simulink library "Airframes"  (Simulink 7.3)
settings: Solver=ode45  StartTime=0.0  StopTime=10.0  RelTol=1e-3
undefined symbols (not defined in the file or in its folder): Vo
libraries: aero_sim_lib x4, simulink x2
(part 2 of 2)

== system Airframes/Cesna A-37/T-37Airframe/Aero. Coef. (Stability Axis)/[C_Y,C_g_L,C_g_N] ==
  u : Inport
  CY_p : Constant  Value=CY_p  OutDataType=fixdt(1, 16)  OutScaling=2^0
  Clm_p : Constant  Value=Clm_p  OutDataType=fixdt(1, 16)  OutScaling=2^0
  Cmm_p : Constant  Value=Cnm_p  OutDataType=fixdt(1, 16)  OutScaling=2^0
  Dot Product : DotProduct  OutDataType=fixdt(1, 16)  OutScaling=2^-10  InputSameDT=on  OutDataTypeStr=Inherit: Inherit via internal rule
  Dot Product1 : DotProduct  OutDataType=fixdt(1, 16)  OutScaling=2^-10  InputSameDT=on  OutDataTypeStr=Inherit: Inherit via internal rule
  Dot Product2 : DotProduct  OutDataType=fixdt(1, 16)  OutScaling=2^-10  InputSameDT=on  OutDataTypeStr=Inherit: Inherit via internal rule
  C_Y : Outport
  C_g_L : Outport  Port=2
  C_g_N : Outport  Port=3
  wires:
  Dot Product2/1 -> C_g_N/1  "C_g_N"
  Dot Product1/1 -> C_g_L/1  "C_g_L"
  Dot Product/1 -> C_Y/1  "C_Y"
  Cmm_p/1 -> Dot Product2/2
  CY_p/1 -> Dot Product/2
  u/1 -> Dot Product/1, Dot Product1/1, Dot Product2/1
  Clm_p/1 -> Dot Product1/2

== system Airframes/Cesna A-37/T-37Airframe/Alpha,Beta,Mach/Dynamic Pressure ==
  V : Inport  OutDataType=sfix(16)  OutScaling=2^0
  Air Density : Inport  Port=2  OutDataType=sfix(16)  OutScaling=2^0
  1/2rhoV^2 : Gain  Gain=1/2  ParameterDataType=sfix(16)  ParameterScaling=2^0  OutDataType=sfix(16)  OutScaling=2^0  SaturateOnIntegerOverflow=on  OutDataTypeStr=Inherit: Same as input  ParamDataTypeStr=Inherit: Same as input
  Product1 : Product  OutDataType=sfix(16)  OutScaling=2^0  SaturateOnIntegerOverflow=on  InputSameDT=on  OutDataTypeStr=Inherit: Same as first input
  Product2 : Product  OutDataType=sfix(16)  OutScaling=2^0  SaturateOnIntegerOverflow=on  InputSameDT=on  OutDataTypeStr=Inherit: Same as first input
  qbar : Outport  OutDataType=sfix(16)  OutScaling=2^0  InitialOutput=0
  wires:
  1/2rhoV^2/1 -> qbar/1
  Product2/1 -> 1/2rhoV^2/1
  Air Density/1 -> Product2/2
  Product1/1 -> Product2/1
  V/1 -> Product1/1, Product1/2

== system Airframes/Cesna A-37/T-37Airframe/Alpha,Beta,Mach/Incidence, Sideslip & Airspeed ==
  Vb : Inport  OutDataType=sfix(16)  OutScaling=2^0
  Airspeed : Math  Operator=sqrt  OutDataType=sfix(16)  OutScaling=2^0  SaturateOnIntegerOverflow=on
  Dot Product : DotProduct  OutDataType=fixdt(1, 16)  OutScaling=2^-10  InputSameDT=on  OutDataTypeStr=Inherit: Inherit via internal rule
  Incidence : Trigonometry  Operator=atan2
  Product : Product  Inputs=*/  OutDataType=sfix(16)  OutScaling=2^0  SaturateOnIntegerOverflow=on  OutDataTypeStr=Inherit: Same as first input
  Sideslip : Trigonometry  Operator=asin
  Subsystem : Subsystem
  Subsystem1 : Subsystem
  Alpha : Outport  OutDataType=sfix(16)  OutScaling=2^0  InitialOutput=0
  Beta : Outport  Port=2  OutDataType=sfix(16)  OutScaling=2^0  InitialOutput=0
  V : Outport  Port=3  OutDataType=sfix(16)  OutScaling=2^0  InitialOutput=0
  wires:
  Product/1 -> Sideslip/1
  Subsystem/1(w) -> Incidence/1
  Subsystem/2(u) -> Incidence/2
  Dot Product/1 -> Airspeed/1
  Airspeed/1 -> Product/2, V/1
  Incidence/1 -> Alpha/1
  Vb/1 -> Subsystem/1(Vb), Subsystem1/1(Vb), Dot Product/1, Dot Product/2
  Sideslip/1 -> Beta/1
  Subsystem1/1(v) -> Product/1

== system Airframes/Cesna A-37/T-37Airframe/Alpha,Beta,Mach/Mach Number ==
  V : Inport  OutDataType=sfix(16)  OutScaling=2^0
  a : Inport  Port=2  OutDataType=sfix(16)  OutScaling=2^0
  Product1 : Product  Inputs=*/  OutDataType=sfix(16)  OutScaling=2^0  SaturateOnIntegerOverflow=on  InputSameDT=on  OutDataTypeStr=Inherit: Same as first input
  Mach : Outport  OutDataType=sfix(16)  OutScaling=2^0
  wires:
  Product1/1 -> Mach/1
  a/1 -> Product1/2
  V/1 -> Product1/1

== system Airframes/Cesna A-37/T-37Airframe/Environment Models/Wind Models ==
  Euler : Inport  OutDataType=sfix(16)  OutScaling=2^0
  Ve : Inport  Port=2  OutDataType=sfix(16)  OutScaling=2^0
  Airspeed : Inport  Port=3  OutDataType=sfix(16)  OutScaling=2^0
  Altitude : Inport  Port=4  OutDataType=sfix(16)  OutScaling=2^0
  DCM : Inport  Port=5  OutDataType=sfix(16)  OutScaling=2^0
  MIL-F-8785C Wind Gust Model (to do) : Subsystem  mask{G_u=on, G_v=on, G_w=on, t_0=100, x_m=10*[b,b,b], v_m=[5,5,5]}
      mask prompts: G_u "Gust in u-axis [G_u]"; G_v "Gust in v-axis [G_v]"; G_w "Gust in w-axis [G_w]"; t_0 "Gust start-time [t_0] (sec):"; x_m "Gust legth x_m=[x_u,x_v,x_w] (m):"; v_m "Gust amplitude v_m=[v_u,v_v,v_w](m/s):"
  MIL-F-8785C Wind Shear Model : Subsystem  mask{phase=Category C (Terminal Flight), u20=6, deg=0}
      mask prompts: phase "Select Flight Phase [phase]"; u20 "Wind Speed at 20 feet above ground [u20] (m/sec)"; deg "Approach Angle of Wind (clock-wise from the North) [deg] (degrees)"
      mask StyleString: popup(Category C (Terminal Flight)|Category A or B (Not Terminal Flight)),edit,edit
  Need Dryden Turbulent Model Block : Constant  Value=[0,0,0]  OutDataType=fixdt(1, 16)  OutScaling=2^0
  Sum : Sum  Inputs=+|+  OutDataType=sfix(16)  OutScaling=2^0  SaturateOnIntegerOverflow=on  InputSameDT=on  OutDataTypeStr=Inherit: Same as first input
  Terminator : Terminator
  Terminator1 : Terminator
  ug,vg,wg : Outport  OutDataType=sfix(16)  OutScaling=2^0
  pg,qg,rg : Outport  Port=2  OutDataType=sfix(16)  OutScaling=2^0
  wires:
  Altitude/1 -> MIL-F-8785C Wind Shear Model/1(h)
  Airspeed/1 -> MIL-F-8785C Wind Gust Model (to do)/1(V(m/s))
  DCM/1 -> MIL-F-8785C Wind Shear Model/2(DCM)
  Sum/1 -> ug,vg,wg/1
  Ve/1 -> Terminator/1
  Euler/1 -> Terminator1/1
  MIL-F-8785C Wind Shear Model/1(v_w) -> Sum/1
  MIL-F-8785C Wind Gust Model (to do)/1(v_w(m/s)) -> Sum/2
  Need Dryden Turbulent Model Block/1 -> pg,qg,rg/1

== system Airframes/Cesna A-37/T-37Airframe/Environment Models/gravity model ==
  h : Inport
  Divide : Product  Inputs=*/  OutDataType=fixdt(1, 16)  OutScaling=2^-10
  Dot Product1 : DotProduct  OutDataType=fixdt(1, 16)  OutScaling=2^-10  InputSameDT=on  OutDataTypeStr=Inherit: Inherit via internal rule
  Model Info : simulink/Model-Wide Utilities/Model Info  SystemSampleTime=-1  InitialBlockCM=None  BlockCM=None  Frame=on  DisplayStringWithTags=g = g_o [R/(R+h)]^2  HorizontalTextAlignment=Center  LeftAlignmentValue=0.5  SourceBlockDiagram=Airframes  TagMaxNumber=20
  R = Radius of Earth (m) : Constant  Value=6356e3  OutDataType=fixdt(1, 16)  OutScaling=2^0
  Sum : Sum  Inputs=|++  OutDataType=fixdt(1, 16)  OutScaling=2^0
  g_o : Gain  Gain=9.80665  ParameterDataType=fixdt(1, 16)  ParameterScaling=2^0  OutDataType=fixdt(1, 16)  OutScaling=2^0
  g : Outport
  wires:
  R = Radius of Earth (m)/1 -> Sum/2, Divide/1
  Sum/1 -> Divide/2
  Divide/1 -> Dot Product1/1, Dot Product1/2
  Dot Product1/1 -> g_o/1
  h/1 -> Sum/1
  g_o/1 -> g/1

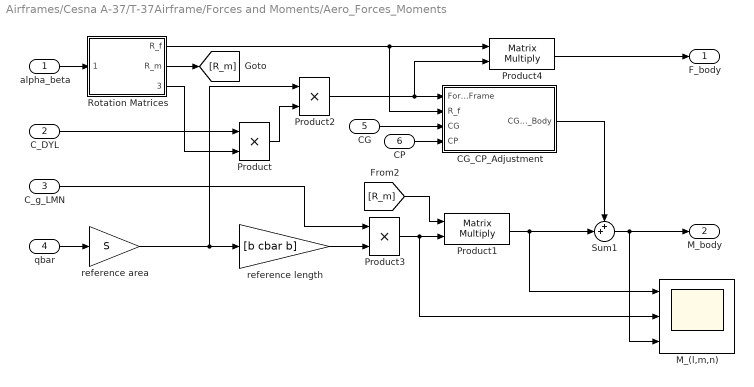
== system Airframes/Cesna A-37/T-37Airframe/Forces and Moments/Aero_Forces_Moments ==
  alpha_beta : Inport
  C_DYL : Inport  Port=2
  C_g_LMN : Inport  Port=3
  qbar : Inport  Port=4
  CG : Inport  Port=5  OutDataType=sfix(16)  OutScaling=2^0
  CP : Inport  Port=6  OutDataType=sfix(16)  OutScaling=2^0
  CG_CP_Adjustment : Subsystem
  M_(l,m,n) : Scope  NumInputPorts=3
      settings: YMin=-5~-5~-5  YMax=5~5~5  SaveName=ScopeData7  SampleInput=on  SampleTime=0.01
  Product : Product  OutDataType=sfix(16)  OutScaling=2^0  SaturateOnIntegerOverflow=on  InputSameDT=on  OutDataTypeStr=Inherit: Same as first input
  Product1 : Product  Multiplication=Matrix(*)  OutDataType=sfix(16)  OutScaling=2^0  RndMeth=Zero
  Product2 : Product  OutDataType=sfix(16)  OutScaling=2^0  SaturateOnIntegerOverflow=on  InputSameDT=on  OutDataTypeStr=Inherit: Same as first input
  Product3 : Product  OutDataType=sfix(16)  OutScaling=2^0  SaturateOnIntegerOverflow=on  InputSameDT=on  OutDataTypeStr=Inherit: Same as first input
  Product4 : Product  Multiplication=Matrix(*)  OutDataType=sfix(16)  OutScaling=2^0  RndMeth=Zero
  Rotation Matrices : Stateflow chart
  Sum1 : Sum  Inputs=++|  OutDataType=sfix(16)  OutScaling=2^0  SaturateOnIntegerOverflow=on  InputSameDT=on  OutDataTypeStr=Inherit: Same as first input
  reference area : Gain  Gain=S  ParameterDataType=sfix(16)  ParameterScaling=2^0  OutDataType=sfix(16)  OutScaling=2^0  SaturateOnIntegerOverflow=on  OutDataTypeStr=Inherit: Same as input  ParamDataTypeStr=Inherit: Same as input
  reference length : Gain  Gain=[b cbar b]  ParameterDataType=sfix(16)  ParameterScaling=2^0  OutDataType=sfix(16)  OutScaling=2^0  SaturateOnIntegerOverflow=on  OutDataTypeStr=Inherit: Same as input  ParamDataTypeStr=Inherit: Same as input
  F_body : Outport
  M_body : Outport  Port=2
  wires:
  alpha_beta/1 -> Rotation Matrices/1(alpha_beta)
  qbar/1 -> reference area/1
  reference area/1 -> reference length/1, Product2/1
  C_DYL/1 -> Product/1
  Rotation Matrices/3(K_adjust) -> Product/2
  reference length/1 -> Product3/2
  C_g_LMN/1 -> Product3/1
  CG/1 -> CG_CP_Adjustment/3(CG)
  CP/1 -> CG_CP_Adjustment/4(CP)
  Rotation Matrices/1(R_f) -> Product4/1, CG_CP_Adjustment/2(R_f)
  Product/1 -> Product2/2
  Product2/1 -> Product4/2, CG_CP_Adjustment/1(Forces_Drag_Frame)
  Product4/1 -> F_body/1
  Rotation Matrices/2(R_m) -> [R_m]
  [R_m] -> Product1/1
  Product3/1 -> M_(l,m,n)/2, Product1/2
  Product1/1 -> M_(l,m,n)/1, Sum1/2
  CG_CP_Adjustment/1(CGP_M_Body) -> Sum1/1
  Sum1/1 -> M_(l,m,n)/3, M_body/1

== system Airframes/Cesna 172P (Skyhawk) Airframe/Alpha,Beta,Mach/Incidence, Sideslip & Airspeed/Subsystem ==
  Vb : Inport  OutDataType=sfix(16)  OutScaling=2^0
  Demux1 : Demux  Outputs=3
  Terminator : Terminator
  w : Outport  OutDataType=sfix(16)  OutScaling=2^0
  u : Outport  Port=2  OutDataType=sfix(16)  OutScaling=2^0
  wires:
  Demux1/1 -> u/1
  Vb/1 -> Demux1/1
  Demux1/2 -> Terminator/1
  Demux1/3 -> w/1

== system Airframes/Cesna 172P (Skyhawk) Airframe/Alpha,Beta,Mach/Incidence, Sideslip & Airspeed/Subsystem1 ==
  Vb : Inport  OutDataType=sfix(16)  OutScaling=2^0
  Demux1 : Demux  Outputs=3
  Terminator : Terminator
  Terminator1 : Terminator
  v : Outport  OutDataType=sfix(16)  OutScaling=2^0
  wires:
  Demux1/2 -> v/1
  Vb/1 -> Demux1/1
  Demux1/3 -> Terminator1/1
  Demux1/1 -> Terminator/1

== system Airframes/Cesna 172P (Skyhawk) Airframe/Environment Models/Wind Models/MIL-F-8785C Wind Gust Model (to do) ==
  V(m/s) : Inport
  Clock : Clock
      settings: Decimation=10
  Constant : Constant  Value=t_0  OutDataType=fixdt(1, 16)  OutScaling=2^0
  Relational Operator : RelationalOperator  LogicOutDataTypeMode=boolean  LogicDataType=fixdt(0, 8)  OutDataTypeStr=boolean
  Triggered Gusts : Subsystem
  v_w(m/s) : Outport
  wires:
  Triggered Gusts/1(v_w) -> v_w(m/s)/1
  V(m/s)/1 -> Triggered Gusts/1(V(m/s))
  Relational Operator/1 -> Triggered Gusts/Enable
  Constant/1 -> Relational Operator/2
  Clock/1 -> Relational Operator/1

== system Airframes/Cesna 172P (Skyhawk) Airframe/Environment Models/Wind Models/MIL-F-8785C Wind Shear Model ==
  h : Inport
  DCM : Inport  Port=2
  MIL-F-8785-Wind Shear Model : Stateflow chart
  v_w : Outport
  wires:
  MIL-F-8785-Wind Shear Model/1(v_w) -> v_w/1
  DCM/1 -> MIL-F-8785-Wind Shear Model/2(DCM)
  h/1 -> MIL-F-8785-Wind Shear Model/1(h)

== system Airframes/Cesna 172P (Skyhawk) Airframe/Forces and Moments/Aero_Forces_Moments/CG_CP_Adjustment ==
  Forces_Drag_Frame : Inport
  R_f : Inport  Port=2
  CG : Inport  Port=3
  CP : Inport  Port=4
  CrossProduct(AXB) : aero_sim_lib/CrossProduct(AXB)  SystemSampleTime=-1
  Product1 : Product  Multiplication=Matrix(*)  OutDataType=sfix(16)  OutScaling=2^0  RndMeth=Zero
  Product2 : Product  Multiplication=Matrix(*)  OutDataType=sfix(16)  OutScaling=2^0  RndMeth=Zero
  Sum : Sum  Inputs=|+-  OutDataType=sfix(16)  OutScaling=2^0  SaturateOnIntegerOverflow=on
  Transpose : Math  Operator=transpose  OutDataType=sfix(16)  OutScaling=2^0  SaturateOnIntegerOverflow=on
  CGP_M_Body : Outport
  wires:
  CrossProduct(AXB)/1 -> Product2/2  "CGP_Moments_Drag_Frame"
  Product2/1 -> CGP_M_Body/1
  CP/1 -> Sum/2
  CG/1 -> Sum/1
  R_f/1 -> Product2/1, Transpose/1  "Rotation_Matrix_Drag_Frame_To_Body_Frame"
  Forces_Drag_Frame/1 -> CrossProduct(AXB)/1
  Product1/1 -> CrossProduct(AXB)/2  "DX_Drag_Frame"
  Sum/1 -> Product1/2  "DX_Body"
  Transpose/1 -> Product1/1

== system Airframes/Cesna A-37/T-37Airframe/Alpha,Beta,Mach/Incidence, Sideslip & Airspeed/Subsystem ==
  Vb : Inport  OutDataType=sfix(16)  OutScaling=2^0
  Demux1 : Demux  Outputs=3
  Terminator : Terminator
  w : Outport  OutDataType=sfix(16)  OutScaling=2^0
  u : Outport  Port=2  OutDataType=sfix(16)  OutScaling=2^0
  wires:
  Demux1/3 -> w/1
  Demux1/2 -> Terminator/1
  Vb/1 -> Demux1/1
  Demux1/1 -> u/1

== system Airframes/Cesna A-37/T-37Airframe/Alpha,Beta,Mach/Incidence, Sideslip & Airspeed/Subsystem1 ==
  Vb : Inport  OutDataType=sfix(16)  OutScaling=2^0
  Demux1 : Demux  Outputs=3
  Terminator : Terminator
  Terminator1 : Terminator
  v : Outport  OutDataType=sfix(16)  OutScaling=2^0
  wires:
  Demux1/1 -> Terminator/1
  Demux1/3 -> Terminator1/1
  Vb/1 -> Demux1/1
  Demux1/2 -> v/1

== system Airframes/Cesna A-37/T-37Airframe/Environment Models/Wind Models/MIL-F-8785C Wind Gust Model (to do) ==
  V(m/s) : Inport
  Clock : Clock
      settings: Decimation=10
  Constant : Constant  Value=t_0  OutDataType=fixdt(1, 16)  OutScaling=2^0
  Relational Operator : RelationalOperator  LogicOutDataTypeMode=boolean  LogicDataType=fixdt(0, 8)  OutDataTypeStr=boolean
  Triggered Gusts : Subsystem
  v_w(m/s) : Outport
  wires:
  Clock/1 -> Relational Operator/1
  Constant/1 -> Relational Operator/2
  Relational Operator/1 -> Triggered Gusts/Enable
  V(m/s)/1 -> Triggered Gusts/1(V(m/s))
  Triggered Gusts/1(v_w) -> v_w(m/s)/1

== system Airframes/Cesna A-37/T-37Airframe/Environment Models/Wind Models/MIL-F-8785C Wind Shear Model ==
  h : Inport
  DCM : Inport  Port=2
  MIL-F-8785-Wind Shear Model : Stateflow chart
  v_w : Outport
  wires:
  h/1 -> MIL-F-8785-Wind Shear Model/1(h)
  DCM/1 -> MIL-F-8785-Wind Shear Model/2(DCM)
  MIL-F-8785-Wind Shear Model/1(v_w) -> v_w/1

== system Airframes/Cesna A-37/T-37Airframe/Forces and Moments/Aero_Forces_Moments/CG_CP_Adjustment ==
  Forces_Drag_Frame : Inport
  R_f : Inport  Port=2
  CG : Inport  Port=3
  CP : Inport  Port=4
  CrossProduct(AXB) : aero_sim_lib/CrossProduct(AXB)  SystemSampleTime=-1
  Product1 : Product  Multiplication=Matrix(*)  OutDataType=sfix(16)  OutScaling=2^0  RndMeth=Zero
  Product2 : Product  Multiplication=Matrix(*)  OutDataType=sfix(16)  OutScaling=2^0  RndMeth=Zero
  Sum : Sum  Inputs=|+-  OutDataType=sfix(16)  OutScaling=2^0  SaturateOnIntegerOverflow=on
  Transpose : Math  Operator=transpose  OutDataType=sfix(16)  OutScaling=2^0  SaturateOnIntegerOverflow=on
  CGP_M_Body : Outport
  wires:
  Transpose/1 -> Product1/1
  Sum/1 -> Product1/2  "DX_Body"
  Product1/1 -> CrossProduct(AXB)/2  "DX_Drag_Frame"
  Forces_Drag_Frame/1 -> CrossProduct(AXB)/1
  R_f/1 -> Transpose/1, Product2/1  "Rotation_Matrix_Drag_Frame_To_Body_Frame"
  CG/1 -> Sum/1
  CP/1 -> Sum/2
  Product2/1 -> CGP_M_Body/1
  CrossProduct(AXB)/1 -> Product2/2  "CGP_Moments_Drag_Frame"

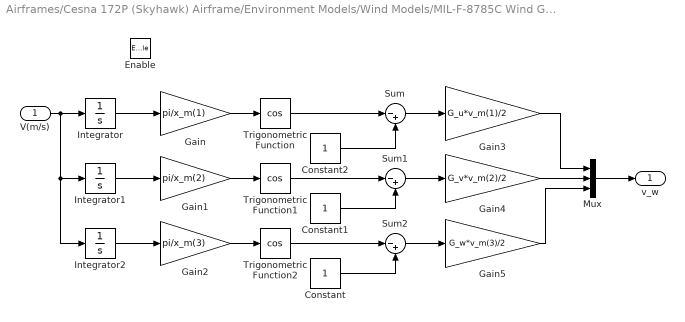
== system Airframes/Cesna 172P (Skyhawk) Airframe/Environment Models/Wind Models/MIL-F-8785C Wind Gust Model (to do)/Triggered Gusts ==
  V(m/s) : Inport
  Enable : EnablePort
  Constant : Constant  OutDataType=fixdt(1, 16)  OutScaling=2^0
  Constant1 : Constant  OutDataType=fixdt(1, 16)  OutScaling=2^0
  Constant2 : Constant  OutDataType=fixdt(1, 16)  OutScaling=2^0
  Gain : Gain  Gain=pi/x_m(1)  ParameterDataType=fixdt(1, 16)  ParameterScaling=2^0  OutDataType=fixdt(1, 16)  OutScaling=2^0
  Gain1 : Gain  Gain=pi/x_m(2)  ParameterDataType=fixdt(1, 16)  ParameterScaling=2^0  OutDataType=fixdt(1, 16)  OutScaling=2^0
  Gain2 : Gain  Gain=pi/x_m(3)  ParameterDataType=fixdt(1, 16)  ParameterScaling=2^0  OutDataType=fixdt(1, 16)  OutScaling=2^0
  Gain3 : Gain  Gain=G_u*v_m(1)/2  ParameterDataType=fixdt(1, 16)  ParameterScaling=2^0  OutDataType=fixdt(1, 16)  OutScaling=2^0
  Gain4 : Gain  Gain=G_v*v_m(2)/2  ParameterDataType=fixdt(1, 16)  ParameterScaling=2^0  OutDataType=fixdt(1, 16)  OutScaling=2^0
  Gain5 : Gain  Gain=G_w*v_m(3)/2  ParameterDataType=fixdt(1, 16)  ParameterScaling=2^0  OutDataType=fixdt(1, 16)  OutScaling=2^0
  Integrator : Integrator  LimitOutput=on  UpperSaturationLimit=x_m(1)  LowerSaturationLimit=0
  Integrator1 : Integrator  LimitOutput=on  UpperSaturationLimit=x_m(2)  LowerSaturationLimit=0
  Integrator2 : Integrator  LimitOutput=on  UpperSaturationLimit=x_m(3)  LowerSaturationLimit=0
  Mux : Mux  Inputs=3
  Sum : Sum  Inputs=|-+  OutDataType=fixdt(1, 16)  OutScaling=2^0
  Sum1 : Sum  Inputs=|-+  OutDataType=fixdt(1, 16)  OutScaling=2^0
  Sum2 : Sum  Inputs=|-+  OutDataType=fixdt(1, 16)  OutScaling=2^0
  Trigonometric Function : Trigonometry  Operator=cos
  Trigonometric Function1 : Trigonometry  Operator=cos
  Trigonometric Function2 : Trigonometry  Operator=cos
  v_w : Outport  OutDataType=fixdt(1, 16)  OutScaling=2^0  InitialOutput=[0,0,0]
  wires:
  Mux/1 -> v_w/1
  Gain5/1 -> Mux/3
  Gain4/1 -> Mux/2
  Gain3/1 -> Mux/1
  Sum1/1 -> Gain4/1
  Sum2/1 -> Gain5/1
  Sum/1 -> Gain3/1
  Constant2/1 -> Sum/2
  Constant1/1 -> Sum1/2
  Constant/1 -> Sum2/2
  Trigonometric Function2/1 -> Sum2/1
  Trigonometric Function1/1 -> Sum1/1
  Trigonometric Function/1 -> Sum/1
  Gain2/1 -> Trigonometric Function2/1
  Integrator2/1 -> Gain2/1
  Gain1/1 -> Trigonometric Function1/1
  Integrator1/1 -> Gain1/1
  Gain/1 -> Trigonometric Function/1
  Integrator/1 -> Gain/1
  V(m/s)/1 -> Integrator2/1, Integrator1/1, Integrator/1

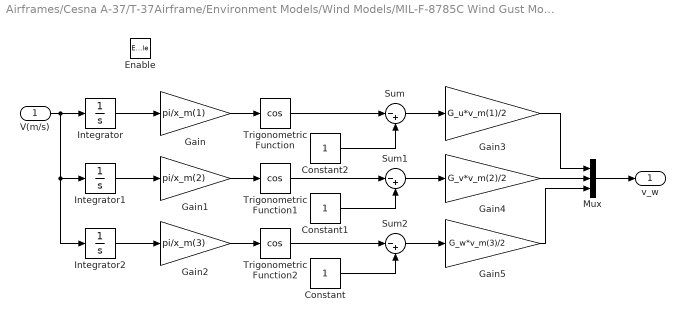
== system Airframes/Cesna A-37/T-37Airframe/Environment Models/Wind Models/MIL-F-8785C Wind Gust Model (to do)/Triggered Gusts ==
  V(m/s) : Inport
  Enable : EnablePort
  Constant : Constant  OutDataType=fixdt(1, 16)  OutScaling=2^0
  Constant1 : Constant  OutDataType=fixdt(1, 16)  OutScaling=2^0
  Constant2 : Constant  OutDataType=fixdt(1, 16)  OutScaling=2^0
  Gain : Gain  Gain=pi/x_m(1)  ParameterDataType=fixdt(1, 16)  ParameterScaling=2^0  OutDataType=fixdt(1, 16)  OutScaling=2^0
  Gain1 : Gain  Gain=pi/x_m(2)  ParameterDataType=fixdt(1, 16)  ParameterScaling=2^0  OutDataType=fixdt(1, 16)  OutScaling=2^0
  Gain2 : Gain  Gain=pi/x_m(3)  ParameterDataType=fixdt(1, 16)  ParameterScaling=2^0  OutDataType=fixdt(1, 16)  OutScaling=2^0
  Gain3 : Gain  Gain=G_u*v_m(1)/2  ParameterDataType=fixdt(1, 16)  ParameterScaling=2^0  OutDataType=fixdt(1, 16)  OutScaling=2^0
  Gain4 : Gain  Gain=G_v*v_m(2)/2  ParameterDataType=fixdt(1, 16)  ParameterScaling=2^0  OutDataType=fixdt(1, 16)  OutScaling=2^0
  Gain5 : Gain  Gain=G_w*v_m(3)/2  ParameterDataType=fixdt(1, 16)  ParameterScaling=2^0  OutDataType=fixdt(1, 16)  OutScaling=2^0
  Integrator : Integrator  LimitOutput=on  UpperSaturationLimit=x_m(1)  LowerSaturationLimit=0
  Integrator1 : Integrator  LimitOutput=on  UpperSaturationLimit=x_m(2)  LowerSaturationLimit=0
  Integrator2 : Integrator  LimitOutput=on  UpperSaturationLimit=x_m(3)  LowerSaturationLimit=0
  Mux : Mux  Inputs=3
  Sum : Sum  Inputs=|-+  OutDataType=fixdt(1, 16)  OutScaling=2^0
  Sum1 : Sum  Inputs=|-+  OutDataType=fixdt(1, 16)  OutScaling=2^0
  Sum2 : Sum  Inputs=|-+  OutDataType=fixdt(1, 16)  OutScaling=2^0
  Trigonometric Function : Trigonometry  Operator=cos
  Trigonometric Function1 : Trigonometry  Operator=cos
  Trigonometric Function2 : Trigonometry  Operator=cos
  v_w : Outport  OutDataType=fixdt(1, 16)  OutScaling=2^0  InitialOutput=[0,0,0]
  wires:
  V(m/s)/1 -> Integrator/1, Integrator1/1, Integrator2/1
  Integrator/1 -> Gain/1
  Gain/1 -> Trigonometric Function/1
  Integrator1/1 -> Gain1/1
  Gain1/1 -> Trigonometric Function1/1
  Integrator2/1 -> Gain2/1
  Gain2/1 -> Trigonometric Function2/1
  Trigonometric Function/1 -> Sum/1
  Trigonometric Function1/1 -> Sum1/1
  Trigonometric Function2/1 -> Sum2/1
  Constant/1 -> Sum2/2
  Constant1/1 -> Sum1/2
  Constant2/1 -> Sum/2
  Sum/1 -> Gain3/1
  Sum2/1 -> Gain5/1
  Sum1/1 -> Gain4/1
  Gain3/1 -> Mux/1
  Gain4/1 -> Mux/2
  Gain5/1 -> Mux/3
  Mux/1 -> v_w/1

== matlab function Cesna A-37/T-37Airframe/Environment Models/Air Properties ==
  data: h input double; T output double; rho output double; g input double; ps output double; a output double
function [T,rho, ps, a] = fcn(h, g)
    %h altitude (meters)
    %g gravity at h (m/s^2)
    R = 8.31432; %J/(mol-Kelvin)
    M = 28.9644; %gm/mol
    To = 288.15; %standard temperature [Kelvin]
    Po = 101325; %standard pressure [Pa]
    L = 6.5; %Kelvin/km
    gamma = 1.4; %Gas constant for air
    T = To - 1.0e-3*L*h;            %Temperature at h
    ps = Po*(T/To)^((g*M)/(R*L));   %Pressure at h
    rho = ps/((1000*R/M)*T);        %Density at h
    a = sqrt(gamma*(R/(M*1e-3))*T); %speed of sound (m/s)

== matlab function Cesna A-37/T-37Airframe/Environment Models/Wind Models/MIL-F-8785C Wind Shear Model/MIL-F-8785-Wind Shear Model ==
  data: h input double; v_w output double; DCM input double; phase parameter double; u20 parameter double; deg parameter double
function v_w = fcn(h, DCM, phase, u20, deg)
%Wind Shear Model Based on
%MIL-F-8785C p. 51
if phase == 1
    z0 = 0.15; %Catagory C Flight Phase (Terminal Flight)
else
    z0 = 2.0;  %Other Flight Phases (Non-Terminal Flight)
end
h = h*3.2808399; %meters to feet
den = log(20/z0);
num = h/z0;
if num < 1
    num = 1;
end
num = log(num);
u_w = u20*num/den;
v_w = DCM*[-u_w*cos(pi*deg/180),-u_w*sin(pi*deg/180),0]';

== matlab function Cesna A-37/T-37Airframe/Forces and Moments/Aero_Forces_Moments/Rotation Matrices ==
  data: C_D_input_axes parameter double; alpha_beta input double; C_g_L_input_axes parameter double; R_f output double; R_m output double; K_adjust output double
function [R_f, R_m, K_adjust] = fcn(C_D_input_axes, alpha_beta, C_g_L_input_axes)
if C_D_input_axes == 1
    R_f=calc_R(alpha_beta(1),0); %stability-to-body
    K_adjust=[-1,1,-1]';
elseif C_D_input_axes == 2
    R_f=calc_R(alpha_beta(1),alpha_beta(2)); %wind-to-body
    K_adjust=[-1,-1,-1]';
else
    R_f=eye(3); %body-to-body
    K_adjust=[1,1,1]';
end
if C_g_L_input_axes == C_D_input_axes
    R_m = R_f;
elseif C_g_L_input_axes == 1
    R_m = calc_R(alpha_beta(1),0); %stability-to-body
elseif C_g_L_input_axes == 2
    R_m = calc_R(alpha_beta(1),alpha_beta(2)); %wind-to-body
else
    R_m=eye(3); %body-to-body
end


function R = calc_R(alpha,beta)
    c_a=cos(alpha);
    c_b=cos(beta);
    s_a=sin(alpha);
    s_b=sin(beta);
    R=[c_a*c_b,-c_a*s_b,-s_a;s_b,c_b,0;s_a*c_b,-s_a*s_b,c_a];

== matlab function Cesna 172P (Skyhawk) Airframe/Environment Models/Air Properties ==
  data: h input double; T output double; rho output double; g input double; ps output double; a output double
function [T,rho, ps, a] = fcn(h, g)
    %h altitude (meters)
    %g gravity at h (m/s^2)
    R = 8.31432; %J/(mol-Kelvin)
    M = 28.9644; %gm/mol
    To = 288.15; %standard temperature [Kelvin]
    Po = 101325; %standard pressure [Pa]
    L = 6.5; %Kelvin/km
    gamma = 1.4; %Gas constant for air
    T = To - 1.0e-3*L*h;            %Temperature at h
    ps = Po*(T/To)^((g*M)/(R*L));   %Pressure at h
    rho = ps/((1000*R/M)*T);        %Density at h
    a = sqrt(gamma*(R/(M*1e-3))*T); %speed of sound (m/s)

== matlab function Cesna 172P (Skyhawk) Airframe/Environment Models/Wind Models/MIL-F-8785C Wind Shear Model/MIL-F-8785-Wind Shear Model ==
  data: h input double; v_w output double; DCM input double; phase parameter double; u20 parameter double; deg parameter double
function v_w = fcn(h, DCM, phase, u20, deg)
%Wind Shear Model Based on
%MIL-F-8785C p. 51
if phase == 1
    z0 = 0.15; %Catagory C Flight Phase (Terminal Flight)
else
    z0 = 2.0;  %Other Flight Phases (Non-Terminal Flight)
end
h = h*3.2808399; %meters to feet
den = log(20/z0);
num = h/z0;
if num < 1
    num = 1;
end
num = log(num);
u_w = u20*num/den;
v_w = DCM*[-u_w*cos(pi*deg/180),-u_w*sin(pi*deg/180),0]';

== matlab function Cesna 172P (Skyhawk) Airframe/Forces and Moments/Aero_Forces_Moments/Rotation Matrices ==
  data: C_D_input_axes parameter double; alpha_beta input double; C_g_L_input_axes parameter double; R_f output double; R_m output double; K_adjust output double
function [R_f, R_m, K_adjust] = fcn(C_D_input_axes, alpha_beta, C_g_L_input_axes)
if C_D_input_axes == 1
    R_f=calc_R(alpha_beta(1),0); %stability-to-body
    K_adjust=[-1,1,-1]';
elseif C_D_input_axes == 2
    R_f=calc_R(alpha_beta(1),alpha_beta(2)); %wind-to-body
    K_adjust=[-1,-1,-1]';
else
    R_f=eye(3); %body-to-body
    K_adjust=[1,1,1]';
end
if C_g_L_input_axes == C_D_input_axes
    R_m = R_f;
elseif C_g_L_input_axes == 1
    R_m = calc_R(alpha_beta(1),0); %stability-to-body
elseif C_g_L_input_axes == 2
    R_m = calc_R(alpha_beta(1),alpha_beta(2)); %wind-to-body
else
    R_m=eye(3); %body-to-body
end


function R = calc_R(alpha,beta)
    c_a=cos(alpha);
    c_b=cos(beta);
    s_a=sin(alpha);
    s_b=sin(beta);
    R=[c_a*c_b,-c_a*s_b,-s_a;s_b,c_b,0;s_a*c_b,-s_a*s_b,c_a];
